simulink model "Task2_Cruise_control_plant_model"  (R2021b)
settings: Solver=VariableStepAuto  StartTime=0.0  StopTime=100  FixedStep=Ts  RelTol=1e-3
values from neighbouring files (symbols this model uses):
  m = 1000    [Task2_Cruise_control_input.m]
settings Model: Creator=vinod  LastModifiedBy=vinod

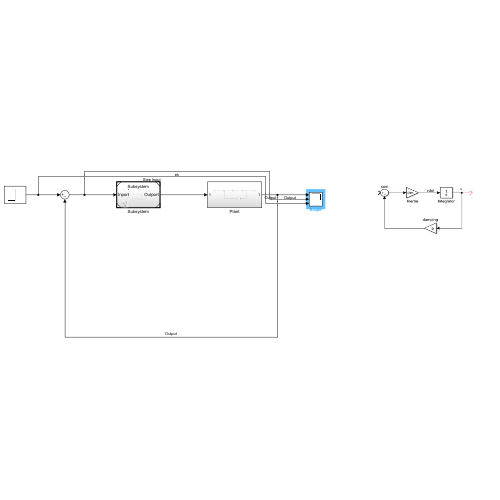
[thumbnail: Simulink's stored preview of the top-level diagram]
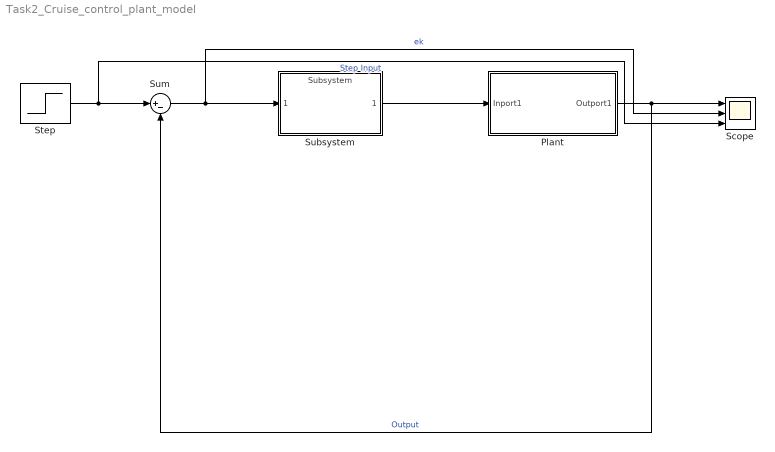
== system Task2_Cruise_control_plant_model ==
  Plant : Subsystem
  Scope : Scope  NumInputPorts=3
  Step : Step  Time=0  After=u  SampleTime=0
  Subsystem : ModelReference  ModelNameDialog=Subsystem  SimulationMode=Normal  ModelReferenceVersion=1.9
  Sum : Sum  Inputs=|+-
  wires:
  Step/1 -> Scope/3, Sum/1  "Step Input"
  Sum/1 -> Subsystem/1, Scope/2  "ek"
  Plant/1(Outport1) -> Sum/2, Scope/1  "Output"
  Subsystem/1 -> Plant/1(Inport1)

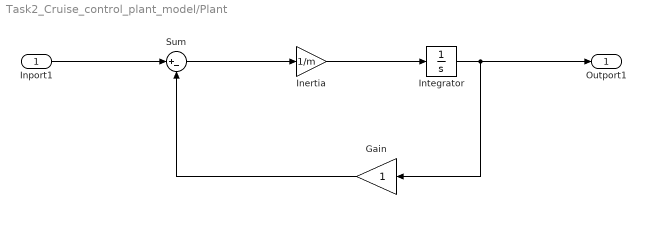
== system Task2_Cruise_control_plant_model/Plant ==
  Inport1 : Inport
  Gain : Gain
  Inertia : Gain  Gain=1/m
  Integrator : Integrator
  Sum : Sum  Inputs=|+-
  Outport1 : Outport
  wires:
  Inertia/1 -> Integrator/1
  Integrator/1 -> Outport1/1, Gain/1
  Sum/1 -> Inertia/1
  Inport1/1 -> Sum/1
  Gain/1 -> Sum/2
